simulink model "testing"  (R2018a)
settings: Solver=VariableStepAuto  StartTime=0.0  StopTime=30  RelTol=1e-3
libraries: libudt x2, simulink x1, sldrtlib x1
settings Model: Creator=Lenovo  LastModifiedBy=Lenovo

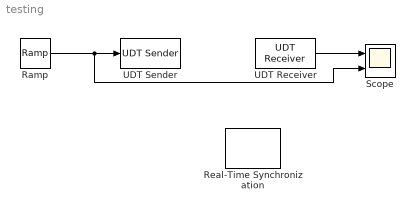
== system testing ==
  Ramp : simulink/Sources/Ramp  slope=0.5  start=0  InitialOutput=0
  Real-Time Synchronization : sldrtlib/Real-Time Synchronization  SampleTime=0.1  MaxMissedTicks=10  ShowMissedTicks=off  YieldWhenWaiting=off
  Scope : Scope  NumInputPorts=2
  UDT Receiver : libudt/UDT Receiver  hostaddress='127.0.0.1'  hostport='2000'  datawidth=1  sampletime=0.01
  UDT Sender : libudt/UDT Sender  hostaddress='127.0.0.1'  hostport='2000'  datawidth=1  sampletime=0.01
  wires:
  UDT Receiver/1 -> Scope/1
  Ramp/1 -> Scope/2, UDT Sender/1
